simulink model "ControlBA"  (R2023b)
settings: Solver=FixedStepDiscrete  StartTime=0.0  StopTime=inf  FixedStep=0.01  RelTol=1e-3  EnableMultiTasking=on
settings Model: ExtModeTrigDuration=2  Creator=Carlos  LastModifiedBy=Carlos
settings OptimizationCC: EnhancedBackFolding=on  PassReuseOutputArgsAs=Individual arguments  ZeroExternalMemoryAtStartup=off  ZeroInternalMemoryAtStartup=off  MaxStackSize=64  OptimizeBlockOrder=speed  DifferentSizesBufferReuse=on  OptimizationCustomize=off  EfficientTunableParamExpr=on
settings DebuggingCC: ParameterTunabilityLossMsg=error
settings HardwareCC: ProdBitPerInt=16  ProdBitPerPointer=16  ProdBitPerSizeT=16  ProdBitPerPtrDiffT=16  ProdLargestAtomicFloat=None  ProdWordSize=8  ProdHWDeviceType=Atmel->AVR
settings SFSimCC: MATLABDynamicMemAlloc=off
settings RTWCC: Description=Embedded Coder  SystemTargetFile=ert.tlc  HardwareBoard=Arduino Mega 2560  TemplateMakefile=ert_default_tmf  Toolchain=Arduino AVR  BuildConfiguration=Faster Runs
settings CodeAppCC: ForceParamTrailComments=on  IgnoreCustomStorageClasses=off  OperatorAnnotations=on  SimulinkDataObjDesc=on  SFDataObjDesc=on  InsertBlockDesc=on
settings ERTTargetCC: SupportContinuousTime=on  SupportVariableSizeSignals=on  ExtModeTransport=3  ExtModeStaticAlloc=on  ExtModeAutomaticAllocSize=off  ExtModeStaticAllocSize=2048  ExtModeMexFile=ext_xcp  ExtModeIntrfLevel=Level2 - Open

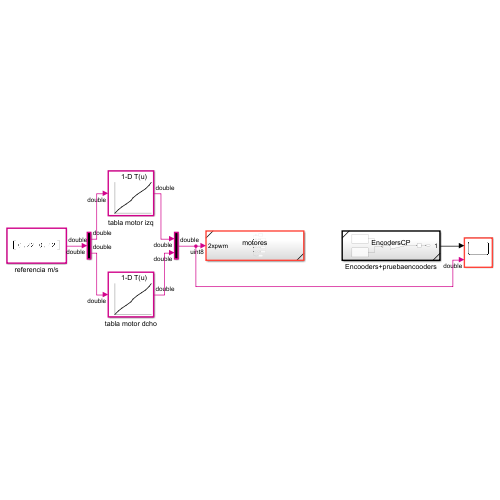
[thumbnail: Simulink's stored preview of the top-level diagram]
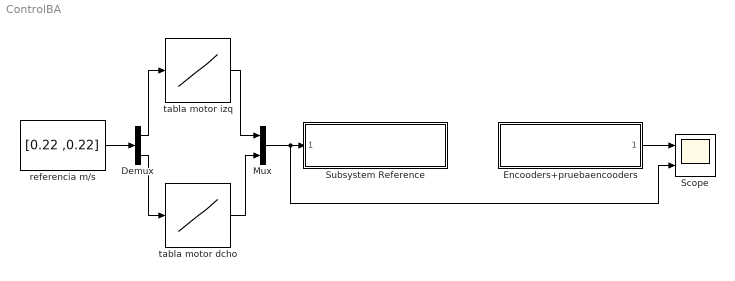
== system ControlBA ==
  Demux : Demux  Outputs=2
  Encooders+pruebaencooders : Subsystem  ReferencedSubsystem=EncodersCP
  Mux : Mux  Inputs=2
  Scope : Scope  NumInputPorts=2
  Subsystem Reference : Subsystem  ReferencedSubsystem=motores
  referencia m/s : Constant  Value=[0.22 ,0.22]
  tabla motor dcho : Lookup_n-D  NumberOfTableDimensions=1  BreakpointsForDimension1=[-0.3816 -0.3094 -0.2372 -0.1547 -0.0516 0 0.0825 0.1753 0.2578 0.33 0.3713]  Table=[-255 -200 -150 -100 -50 0 50 100 150 200 255]  InternalRulePriority=Speed  RndMeth=Simplest
  tabla motor izq : Lookup_n-D  NumberOfTableDimensions=1  BreakpointsForDimension1=[-0.3816 -0.3094 -0.2372 -0.1547 -0.0516 0 0.0825 0.1753 0.2578 0.33 0.3713]  Table=[-255 -200 -150 -100 -50 0 50 100 150 200 255]  InternalRulePriority=Speed  RndMeth=Simplest
  wires:
  Encooders+pruebaencooders/1 -> Scope/1
  referencia m/s/1 -> Demux/1
  Demux/1 -> tabla motor izq/1
  Demux/2 -> tabla motor dcho/1
  Mux/1 -> Scope/2, Subsystem Reference/1
  tabla motor izq/1 -> Mux/1
  tabla motor dcho/1 -> Mux/2
